simulink model "BatteryFastCharging"  (R2026a)
settings: Solver=ode23t  StopTime=p.Duration  MaxStep=1  RelTol=1e-5  AbsTol=1e-7
InitFcn:
  | addpath(fullfile(fileparts(get_param(bdroot,'FileName')),'matlab'));
model workspace (MAT data in the model file):
  logNames = {'time_s', 'current_charge_A', 'voltage_V', 'soc', 'core_K', 'surface_K', 'anode_potential_V', 'anode_surface_mol_m3', 'electrolyte_min_mol_m3', 'internal_soc', 'fault', 'sei_m', 'irreversible_plating_mol', 'reversible_plating_mol', 'complete', 'stop_after_settling', 'termination_reason', 'command_current_A', 'thermal_limit_A', 'anode_limit_A', 'electrolyte_limit_A', 'requested_current_A', 'binding_limiter', 'aging_enabled', 'characterization_replay'}
  p.Q_Ah = 5
  p.SOC0 = 0.2
  p.SOCtarget = 0.8
  p.T0 = 298.15
  p.Tamb = 298.15
  p.Vcontrol = 4.195
  p.Vmax = 4.2
  p.Tmax = 318.15
  p.Imax = 7.5
  p.AnodePotentialMin = 0.02
  p.ElectrolyteMin = 100
  p.Ts = 0.5
  p.Istages = [2.5 2.5 2.5 2.5]
  p.SOCswitch = [0.4 0.6 0.7]
  p.Duration = 12000
  p.Shells = 12
  p.LayersAnode = 12
  p.LayersSeparator = 12
  p.LayersCathode = 12
  p.UseExternalCurrent = 0
  p.InputCurrent = [0  0; 24000  0]
  p.EnableAging = 0
  p.InitialSEI = 5e-09
  p.CharacterizationReplay = 0
  p.StopOnTarget = 1
  p.ImaxDischarge = 7.5
  p.ActuatorTau = 2
  p.ThermalGain = 2
  p.ThermalSoftMargin = 1
  p.AnodeGain = 100
  p.AnodeFaultMin = -0.005
  p.ElectrolyteGain = 0.02
  p.ElectrolyteSoftMargin = 100
  p.VoltageFaultMargin = 0
  p.TemperatureFaultMargin = 0
  p.VoltageMin = 2
  p.SOCmin = 0
  p.DiagnosticVmax = 4.25
  p.DiagnosticVmin = 2
  p.DiagnosticTmax = 333.15
  p.DiagnosticCeMin = 1
  p.DiagnosticAnodeMin = -0.05
  p.ShutdownCurrentTolerance = 0.01
  p.ShutdownMinTime = 0.5
  p.ShutdownMaxTime = 20
  p.MaxStep = 1
  p.RelTol = 1e-05
  p.AbsTol = 1e-07
  p.RLsampleTime = 10
  p.ThicknessAnode = 8.52e-05
  p.ThicknessSeparator = 1.2e-05
  p.ThicknessCathode = 7.56e-05
  p.ElectrodePlateArea = 0.1027
  p.ParticleRadiusAnode = 5.86e-06
  p.ParticleRadiusCathode = 5.22e-06
  p.ActiveMaterialVolumeFractionAnode = 0.75
  p.ActiveMaterialVolumeFractionCathode = 0.665
  p.MaximumConcentrationAnode = 33133
  p.MaximumConcentrationCathode = 63104
  p.MinimumStoichiometryAnode = 0.0263457902706
  p.MaximumStoichiometryAnode = 0.910618046652
  p.MinimumStoichiometryCathode = 0.263845224591
  p.MaximumStoichiometryCathode = 0.85397467463
  p.ActiveMaterialDiffusionCoefficientAnode = 3.3e-14
  p.ActiveMaterialDiffusionCoefficientCathode = 4e-15
  p.ConductivityAnode = 215
  p.ConductivityCathode = 0.18
  p.CurrentCollectorResistance = 0
  p.ElectrolyteVolumeFractionAnode = 0.25
  p.ElectrolyteVolumeFractionSeparator = 0.47
  p.ElectrolyteVolumeFractionCathode = 0.335
  p.ElectrolyteConductivity = 0.9487
  p.ElectrolyteDiffusionCoefficient = 1.7694e-10
  p.BruggemanExponentAnode = 1.5
  p.BruggemanExponentSeparator = 1.5
  p.BruggemanExponentCathode = 1.5
  p.TransferenceNumber = 0.2594
  p.ChargeTransferRateAnode = 6.71604673749e-12
  p.ChargeTransferRateCathode = 3.54458022256e-11
  p.ArrheniusReferenceTemperature = 298.15
  p.ActiveMaterialDiffusionActivationEnergyAnode = 1e-06
  p.ActiveMaterialDiffusionActivationEnergyCathode = 1e-06
  p.ElectrolyteDiffusionActivationEnergy = 1e-06
  p.ElectrolyteConductivityActivationEnergy = 1e-06
  p.ConductivityActivationEnergyAnode = 1e-06
  p.ConductivityActivationEnergyCathode = 1e-06
  p.ChargeTransferActivationEnergyAnode = 35000
  p.ChargeTransferActivationEnergyCathode = 17800
  p.BatteryThermalMass = 42.7752981275
  p.Csurface = 8
  p.RcoreSurface = 1.5
  p.RsurfaceAmbient = 6
  p.Sto = [0.001 0.00266611018364 0.00433222036728 0.00599833055092 0.00766444073456 0.0093305509182 0.0109966611018 0.0126627712855 0.0143288814691 0.0159949916528 0.0176611018364 0.01932721202 ... (600 elements, 600x1)]
  p.Un = [2.30713653173 2.18632839865 2.07318676163 1.96722472974 1.86798629583 1.77504437364 1.68799895927 1.6064754091 1.53012282672 1.4586125519 1.39163674522 1.32890706202 ... (600 elements, 600x1)]
  p.Up = [4.67769531267 4.6763377305 4.67497967199 4.673621114 4.67226203229 4.67090240146 4.66954219491 4.66818138474 4.66681994175 4.66545783534 4.66409503344 4.66273150246 ... (600 elements, 600x1)]
  p.ProfileData = [0  2.5  2.5  2.5  2.5; 24000  2.5  2.5  2.5  2.5]
values from neighbouring files (symbols this model uses):
  p = project_parameters()    [additional_validation.m]    (also in aging_study.m = project_parameters();p.EnableAging=true; battery_diagnostics.m; build_report.m; evaluate_profile_selection.m)
libraries: fl_lib x6, nesl_utility x2, BatteryCurrentManagement x1, batt_lib x1
settings Model: Creator=venum  LastModifiedBy=venum

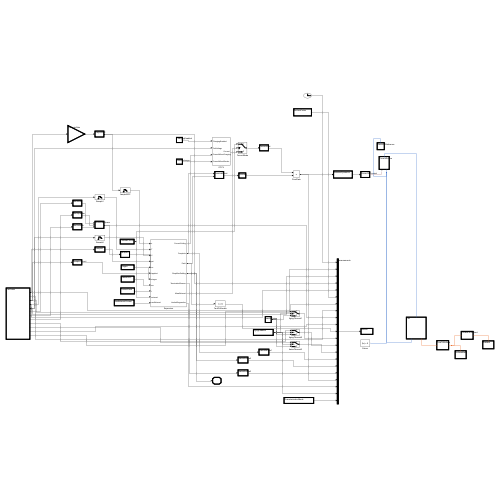
[thumbnail: Simulink's stored preview of the top-level diagram]
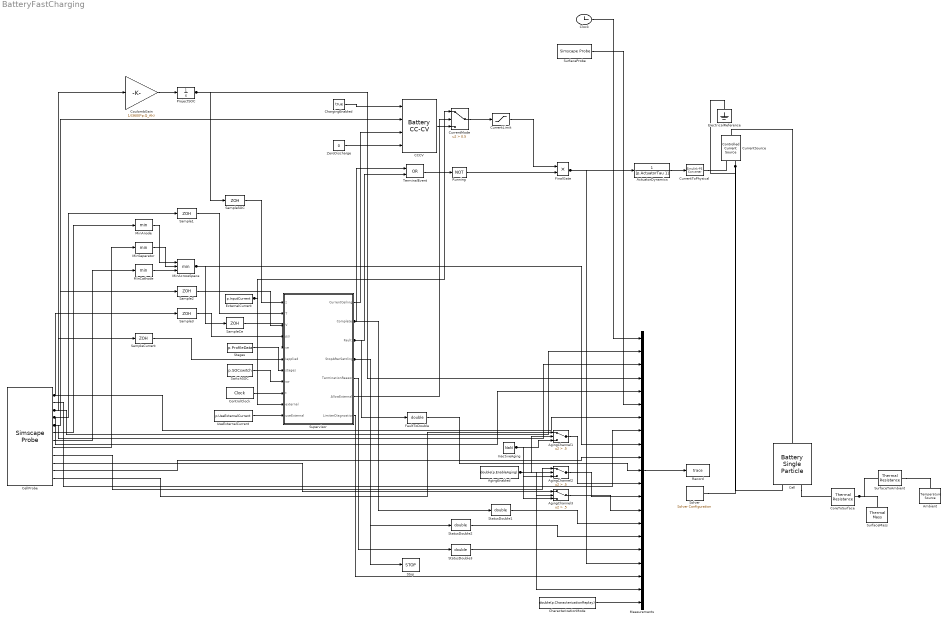
== system BatteryFastCharging ==
  ActuatorDynamics : TransferFcn  Numerator=1  Denominator=[p.ActuatorTau 1]
  AgingChannel1 : Switch  Criteria=u2 > Threshold  Threshold=.5  SaturateOnIntegerOverflow=off  InputSameDT=off
  AgingChannel2 : Switch  Criteria=u2 > Threshold  Threshold=.5  SaturateOnIntegerOverflow=off  InputSameDT=off
  AgingChannel3 : Switch  Criteria=u2 > Threshold  Threshold=.5  SaturateOnIntegerOverflow=off  InputSameDT=off
  AgingEnabled : Constant  Value=double(p.EnableAging)
  Ambient : fl_lib/Thermal/Thermal Sources/Temperature Source  temperature=p.Tamb K
  CCCV : BatteryCurrentManagement/Battery CC-CV  MinMaxFlag=off  MaxCellVoltage=p.Vcontrol  Kp=20  Ki=2  Kaw=1  Kt=1  Ts=p.Ts
  Cell : batt_lib/Cells/Electrochemical/Battery Single Particle  ExtrapolationMethod=simscape.enum.extrapolation.nearest  ThicknessAnode=p.ThicknessAnode m  ElectrolyteLayerCountAnode=p.LayersAnode  ThicknessSeparator=p.ThicknessSeparator m  ElectrolyteLayerCountSeparator=p.LayersSeparator  ThicknessCathode=p.ThicknessCathode m  ElectrolyteLayerCountCathode=p.LayersCathode  ElectrodePlateArea=p.ElectrodePlateArea m^2  ParticleRadiusAnode=p.ParticleRadiusAnode m  ShellCountAnode=p.Shells  ParticleRadiusCathode=p.ParticleRadiusCathode m  ShellCountCathode=p.Shells  ActiveMaterialVolumeFractionAnode=p.ActiveMaterialVolumeFractionAnode  ActiveMaterialVolumeFractionCathode=p.ActiveMaterialVolumeFractionCathode  StoichiometryBreakpointsSpecification=simscape.battery.enum.cells.electrochemical.StoichiometryBreakpointsSpecification.absolute  NormalizedStoichiometryBreakpoints=linspace(0.025, 0.975, 39)  OpenCircuitPotentialAnode=[.435; .325; .259; .221; .204; .194; .179; .166; .155; .145; .137; .131; .128; .127; .126; .125; .124; .123; .122; .121; .118; .117; .112; .109; .105; .1; .098; .095; .094; .093; .091; .09; .089; .088; .087; .086; .085; .084; .083] V  OpenCircuitPotentialCathode=[3.598; 3.53; 3.494; 3.474; 3.46; 3.455; 3.454; 3.453; 3.4528; 3.4526; 3.4524; 3.452; 3.4518; 3.4516; 3.4514; 3.4512; 3.451; 3.4508; 3.4506; 3.4503; 3.45; 3.4498; 3.4495; 3.4493; 3.449; 3.4488; 3.4486; 3.4484; 3.4482; 3.4479; 3.4477; 3.4475; 3.4473; 3.447; 3.4468; 3.4466; 3.4464; 3.4462; 3.4458] V  AbsoluteStoichiometryBreakpointsAnode=p.Sto  OpenCircuitPotentialAbsoluteAnode=p.Un V  AbsoluteStoichiometryBreakpointsCathode=p.Sto  OpenCircuitPotentialAbsoluteCathode=p.Up V  MaximumConcentrationAnode=p.MaximumConcentrationAnode mol/m^3  MaximumStoichiometryAnode=p.MaximumStoichiometryAnode  MinimumStoichiometryAnode=p.MinimumStoichiometryAnode  MaximumConcentrationCathode=p.MaximumConcentrationCathode mol/m^3  MaximumStoichiometryCathode=p.MaximumStoichiometryCathode  MinimumStoichiometryCathode=p.MinimumStoichiometryCathode  ActiveMaterialDiffusionCoefficientAnode=p.ActiveMaterialDiffusionCoefficientAnode m^2/s  ActiveMaterialDiffusionCoefficientCathode=p.ActiveMaterialDiffusionCoefficientCathode m^2/s  ConductivityAnode=p.ConductivityAnode S/m  ConductivityCathode=p.ConductivityCathode S/m  CurrentCollectorResistance=p.CurrentCollectorResistance Ohm  ElectrolyteVolumeFractionAnode=p.ElectrolyteVolumeFractionAnode  ElectrolyteVolumeFractionSeparator=p.ElectrolyteVolumeFractionSeparator  ElectrolyteVolumeFractionCathode=p.ElectrolyteVolumeFractionCathode  ElectrolyteConductivity=p.ElectrolyteConductivity S/m  BruggemanExponentAnode=p.BruggemanExponentAnode  BruggemanExponentSeparator=p.BruggemanExponentSeparator  BruggemanExponentCathode=p.BruggemanExponentCathode  TransferenceNumber=p.TransferenceNumber  ElectrolyteDiffusionCoefficient=p.ElectrolyteDiffusionCoefficient m^2/s  ChargeTransferRateAnode=p.ChargeTransferRateAnode m^(5/2)/(mol^(1/2)*s)  ChargeTransferRateCathode=p.ChargeTransferRateCathode m^(5/2)/(mol^(1/2)*s)  BatteryThermalMass=p.BatteryThermalMass J/K  ArrheniusReferenceTemperature=p.ArrheniusReferenceTemperature K  ActiveMaterialDiffusionActivationEnergyAnode=p.ActiveMaterialDiffusionActivationEnergyAnode J/mol  ActiveMaterialDiffusionActivationEnergyCathode=p.ActiveMaterialDiffusionActivationEnergyCathode J/mol  ElectrolyteDiffusionActivationEnergy=p.ElectrolyteDiffusionActivationEnergy J/mol  ConductivityActivationEnergyAnode=p.ConductivityActivationEnergyAnode J/mol  ConductivityActivationEnergyCathode=p.ConductivityActivationEnergyCathode J/mol  ElectrolyteConductivityActivationEnergy=p.ElectrolyteConductivityActivationEnergy J/mol  ChargeTransferActivationEnergyAnode=p.ChargeTransferActivationEnergyAnode J/mol  ChargeTransferActivationEnergyCathode=p.ChargeTransferActivationEnergyCathode J/mol  InnerSEIMethod=simscape.battery.enum.cells.electrochemical.InnerSEIMethod.none  MolarVolumeInnerSEI=9.585e-5 m^3/mol  DiffusionCoefficientInnerSEI=1e-20 m^2/s  StoichiometricCoefficientInnerSEI=2  DiffusionActivationEnergyInnerSEI=1e-6 J/mol  ConductivityInnerSEI=5e-6 S/m  ConductivityActivationEnergyInnerSEI=39000 J/mol  PlatingMethod=simscape.battery.enum.cells.electrochemical.PlatingMethod.none  ExchangeCurrentDensityPlating=3E-4 A/m^2  ActivationEnergyPlating=3000 J/mol  ReversibilityFactorPlating=0.5  batteryCurrent_specify=off  batteryCurrent_priority=None  batteryCurrent=0 A  batteryCurrent_nominal_specify=off  batteryCurrent_nominal_value=1  batteryCurrent_nominal_unit=A  batteryVoltage_specify=off  batteryVoltage_priority=None  batteryVoltage=0 V  batteryVoltage_nominal_specify=off  batteryVoltage_nominal_value=1  batteryVoltage_nominal_unit=V  averageElectrolyteConcentration_specify=on  averageElectrolyteConcentration_priority=High  averageElectrolyteConcentration=1000 mol/m^3  averageElectrolyteConcentration_nominal_specify=off  averageElectrolyteConcentration_nominal_value=1  averageElectrolyteConcentration_nominal_unit=mol/m^3  stateOfCharge_specify=on  stateOfCharge_priority=High  stateOfCharge=p.SOC0  stateOfCharge_nominal_specify=off  stateOfCharge_nominal_value=1  stateOfCharge_nominal_unit=1  batteryTemperature_specify=on  batteryTemperature_priority=High  batteryTemperature=p.T0 K  batteryTemperature_nominal_specify=off  batteryTemperature_nominal_value=1  batteryTemperature_nominal_unit=K  thicknessSEI_specify=on  thicknessSEI_priority=High  thicknessSEI=p.InitialSEI m  thicknessSEI_nominal_specify=off  thicknessSEI_nominal_value=1  thicknessSEI_nominal_unit=m  reversiblePlatedMaterial_specify=off  reversiblePlatedMaterial_priority=High  reversiblePlatedMaterial=0 mol  reversiblePlatedMaterial_nominal_specify=off  reversiblePlatedMaterial_nominal_value=1  reversiblePlatedMaterial_nominal_unit=mol  irreversiblePlatedMaterial_specify=off  irreversiblePlatedMaterial_priority=High  irreversiblePlatedMaterial=0 mol  irreversiblePlatedMaterial_nominal_specify=off  irreversiblePlatedMaterial_nominal_value=1  irreversiblePlatedMaterial_nominal_unit=mol  power_dissipated_specify=off  power_dissipated_priority=None  power_dissipated=0 W  power_dissipated_nominal_specify=off  power_dissipated_nominal_value=1  power_dissipated_nominal_unit=W  heatGenerationRate_specify=off  heatGenerationRate_priority=None  heatGenerationRate=0 W  heatGenerationRate_nominal_specify=off  heatGenerationRate_nominal_value=1  heatGenerationRate_nominal_unit=W
  CellProbe : SimscapeProbe  BoundBlock=1  Variables="{\"anodeElectrolyteOverpotential\":{\"Probing\":\"ON\"},\"anodeModel.surfaceConcentration\":{\"Probing\":\"ON\"},\"batteryCurrent\":{\"Probing\":\"ON\"},\"batteryTemperature\":{\"Probing\":\"ON\"},\"batteryVoltage\":{\"Probing\":\"ON\"},\"electrolyteModel.concentrationAnode\":{\"Probing\":\"ON\"},\"electrolyteModel.concentrationCathode\":{\"Probing\":\"ON\"},\"electrolyteModel.concentrationSeparator\":{\"Probing\":\"ON\"},\"irreversiblePlatedMaterial\":{\"Probing\":\"ON\"},\"reversiblePlatedMaterial\":{\"Probing\":\"ON\"},\"stateOfCharge\":{\"Probing\":\"ON\"},\"thicknessSEI\":{\"Probing\":\"ON\"}}"
  CharacterizationMode : Constant  Value=double(p.CharacterizationReplay)
  ChargingEnabled : Constant  Value=true  OutDataTypeStr=boolean
  Clock : Clock
  ControlClock : DigitalClock  SampleTime=p.Ts
  CoreToSurface : fl_lib/Thermal/Thermal Elements/Thermal Resistance  resistance=p.RcoreSurface K/W  T_specify=off  T_priority=None  T=0 K  T_nominal_specify=off  T_nominal_value=1  T_nominal_unit=K  Q_specify=off  Q_priority=None  Q=0 W  Q_nominal_specify=off  Q_nominal_value=1  Q_nominal_unit=W
  CoulombGain : Gain  Gain=1/(3600*p.Q_Ah)
  CurrentLimit : Saturate  UpperLimit=p.Imax  LowerLimit=-p.ImaxDischarge
  CurrentMode : Switch  Criteria=u2 > Threshold  Threshold=0.5  SaturateOnIntegerOverflow=off  InputSameDT=off
  CurrentSource : fl_lib/Electrical/Electrical Sources/Controlled Current Source
  CurrentToPhysical : nesl_utility/Simulink-PS Converter  PhysicalDomain=network_engine_domain  SubClassName=ps_input  LeftPortType=input  RightPortType=output  PseudoPeriodic=off  Frequencies=[]  NoiseDistribution=none  NoiseParameters=[]  Unit=A  AffineConversion=off  FilteringAndDerivatives=provide  SimscapeFilterOrder=1  InputFilterTimeConstant=0.001  UdotUserProvided=0
  ElectricalReference : fl_lib/Electrical/Electrical Elements/Electrical Reference
  ExternalCurrent : FromWorkspace  VariableName=p.InputCurrent  SampleTime=p.Ts
  FaultToDouble : DataTypeConversion  OutDataTypeStr=double  SaturateOnIntegerOverflow=off  RndMeth=Floor
  FinalGate : Product
  InactiveAging : Constant  Value=NaN
  Measurements : Mux  Inputs=21
  MinAcrossSpace : MinMax  Inputs=3
  MinAnode : MinMax
  MinCathode : MinMax
  MinSeparator : MinMax
  ProjectSOC : Integrator  InitialCondition=p.SOC0
  Record : ToWorkspace  VariableName=trace  SampleTime=-1
  Running : Logic  Operator=NOT  AllPortsSameDT=off  OutDataTypeStr=boolean
  Sample1 : ZeroOrderHold  SampleTime=p.Ts
  Sample2 : ZeroOrderHold  SampleTime=p.Ts
  Sample3 : ZeroOrderHold  SampleTime=p.Ts
  SampleCe : ZeroOrderHold  SampleTime=p.Ts
  SampleCurrent : ZeroOrderHold  SampleTime=p.Ts
  SampleSOC : ZeroOrderHold  SampleTime=p.Ts
  Solver : nesl_utility/Solver Configuration  PhysicalDomain=network_engine_domain  SubClassName=solver  LeftPortType=input  RightPortType=generic  Tones=[]  Harmonics=[]  SimulateNoise=off  Profile=off  UseLocalSampling=off  EnableSwitchedLinearOptims=on  FrequencyDomain=off  UseCCode=off  RelTol=0.001  AbsTol=0.001  MinStep=1e-09  ToWorkspace=off  RevertToSquareIcSolve=off  NumHomotopyIterations=100  PhasorMode=off  PhasorModeNumHarmonics=1  ConsistencySolver=NEWTON_XTOL_AFTER_FTOL  CanonicalOrdering=CANONICAL  OptimizeIntermediates=OPTIMIZED  IndexReductionMethod=DerivativeReplacement  DoDC=off  ResidualTolerance=1e-09  ConsistencyTolSource=GLOBAL  ConsistencyAbsTol=0.001  ConsistencyRelTol=0.001  ConsistencyTolFactor=0.001  UseLocalSolver=off  LocalSolverChoice=NE_BACKWARD_EULER_ADVANCER  ResolveIndetEquations=on  FunctionEvalNumThread=1  LocalSolverSampleTime=0.001  DoFixedCost=off  MaxNonlinIter=3  MaxModeIter=2  ComputeImpulses=off  ImpulseIterations=2  LinearAlgebra=auto  LinearAlgebraNumThread=0  EquationFormulation=NE_TIME_EF  DelaysMemoryBudget=1024  AutomaticFiltering=on  FilteringTimeConstant=0.001  PartitionStorageMethod=AS_NEEDED  PartitionMemoryBudget=1024  PartitionMethod=ROBUST  MultibodyUseLocalSolver=off  MultibodyLocalSolverChoice=ODE1  MultibodyLocalSolverSampleTime=0.001
  Stages : FromWorkspace  VariableName=p.ProfileData  SampleTime=p.Ts
  StatusDouble1 : DataTypeConversion  OutDataTypeStr=double  SaturateOnIntegerOverflow=off  RndMeth=Floor
  StatusDouble2 : DataTypeConversion  OutDataTypeStr=double  SaturateOnIntegerOverflow=off  RndMeth=Floor
  StatusDouble3 : DataTypeConversion  OutDataTypeStr=double  SaturateOnIntegerOverflow=off  RndMeth=Floor
  Stop : Stop
  Supervisor : Subsystem
  SurfaceMass : fl_lib/Thermal/Thermal Elements/Thermal Mass  mass_type=foundation.enum.constant_variable.constant  mass=1 kg  sp_heat=p.Csurface J/(K*kg)  mass_min=1e-6 kg  num_ports=foundation.enum.numPorts2.one  m_specify=off  m_priority=High  m=1 kg  m_nominal_specify=off  m_nominal_value=1  m_nominal_unit=kg  T_specify=on  T_priority=High  T=p.T0 K  T_nominal_specify=off  T_nominal_value=1  T_nominal_unit=K  Q_specify=off  Q_priority=None  Q=0 W  Q_nominal_specify=off  Q_nominal_value=1  Q_nominal_unit=W
  SurfaceProbe : SimscapeProbe  BoundBlock=8  Variables="{\"T\":{\"Probing\":\"ON\"}}"
  SurfaceToAmbient : fl_lib/Thermal/Thermal Elements/Thermal Resistance  resistance=p.RsurfaceAmbient K/W  T_specify=off  T_priority=None  T=0 K  T_nominal_specify=off  T_nominal_value=1  T_nominal_unit=K  Q_specify=off  Q_priority=None  Q=0 W  Q_nominal_specify=off  Q_nominal_value=1  Q_nominal_unit=W
  SwitchSOC : Constant  Value=p.SOCswitch
  TerminalEvent : Logic  Operator=OR  AllPortsSameDT=off  OutDataTypeStr=boolean
  UseExternalCurrent : Constant  Value=p.UseExternalCurrent
  ZeroDischarge : Constant  Value=0
  wires:
  CellProbe/8 -> MinSeparator/1
  CellProbe/1 -> Sample3/1, Measurements/7
  CellProbe/2 -> Measurements/8
  CellProbe/3 -> Measurements/2, CoulombGain/1, SampleCurrent/1
  CellProbe/4 -> Sample1/1, Measurements/5
  CellProbe/5 -> Sample2/1, CCCV/2, Measurements/3
  Supervisor/5(TerminationReason) -> StatusDouble3/1
  Sample2/1 -> Supervisor/3(V)
  CellProbe/6 -> MinAnode/1
  CellProbe/7 -> MinCathode/1
  AgingChannel1/1 -> Measurements/12
  CellProbe/9 -> AgingChannel2/1
  TerminalEvent/1 -> Running/1
  CellProbe/10 -> AgingChannel3/1
  Supervisor/2(Complete) -> StatusDouble1/1, TerminalEvent/1
  CellProbe/11 -> Measurements/10
  CellProbe/12 -> AgingChannel1/1
  CCCV/1 -> CurrentMode/3
  CoulombGain/1 -> ProjectSOC/1
  AgingChannel2/1 -> Measurements/13
  AgingEnabled/1 -> Measurements/20, AgingChannel1/2, AgingChannel2/2, AgingChannel3/2
  ExternalCurrent/1 -> CurrentMode/1, Supervisor/10(external)
  MinAnode/1 -> MinAcrossSpace/1
  MinSeparator/1 -> MinAcrossSpace/2
  MinCathode/1 -> MinAcrossSpace/3
  SampleCurrent/1 -> Supervisor/6(Iapplied)
  ProjectSOC/1 -> Measurements/4, SampleSOC/1
  Sample1/1 -> Supervisor/2(T)
  MinAcrossSpace/1 -> Measurements/9, SampleCe/1
  Supervisor/6(AllowExternal) -> CurrentMode/2
  Sample3/1 -> Supervisor/4(psi)
  ZeroDischarge/1 -> CCCV/4
  SampleSOC/1 -> Supervisor/1(z)
  SampleCe/1 -> Supervisor/5(ce)
  CurrentLimit/1 -> FinalGate/1
  Stages/1 -> Supervisor/7(stages)
  SwitchSOC/1 -> Supervisor/8(sw)
  ControlClock/1 -> Supervisor/9(t)
  UseExternalCurrent/1 -> Supervisor/11(useExternal)
  StatusDouble2/1 -> Measurements/16
  ChargingEnabled/1 -> CCCV/1
  Supervisor/1(CurrentCeiling) -> CCCV/3
  Clock/1 -> Measurements/1
  Supervisor/3(Fault) -> TerminalEvent/2, FaultToDouble/1
  Supervisor/4(StopAfterSettling) -> Stop/1, StatusDouble2/1
  Supervisor/7(LimiterDiagnostics) -> Measurements/19
  FaultToDouble/1 -> Measurements/11
  CurrentMode/1 -> CurrentLimit/1
  Running/1 -> FinalGate/2
  CharacterizationMode/1 -> Measurements/21
  StatusDouble3/1 -> Measurements/17
  InactiveAging/1 -> AgingChannel1/3, AgingChannel2/3, AgingChannel3/3
  StatusDouble1/1 -> Measurements/15
  SurfaceProbe/1 -> Measurements/6
  FinalGate/1 -> ActuatorDynamics/1, Measurements/18
  AgingChannel3/1 -> Measurements/14
  ActuatorDynamics/1 -> CurrentToPhysical/1
  Measurements/1 -> Record/1
  connections:
  CurrentToPhysical/RConn1 -- CurrentSource/RConn1
  CoreToSurface/RConn1 -- SurfaceMass/LConn1 -- SurfaceToAmbient/LConn1
  Cell/RConn2 -- CoreToSurface/LConn1
  CurrentSource/LConn1 -- Cell/LConn1
  Solver/RConn1 -- ElectricalReference/LConn1 -- Cell/RConn1 -- CurrentSource/RConn2
  SurfaceToAmbient/RConn1 -- Ambient/LConn1

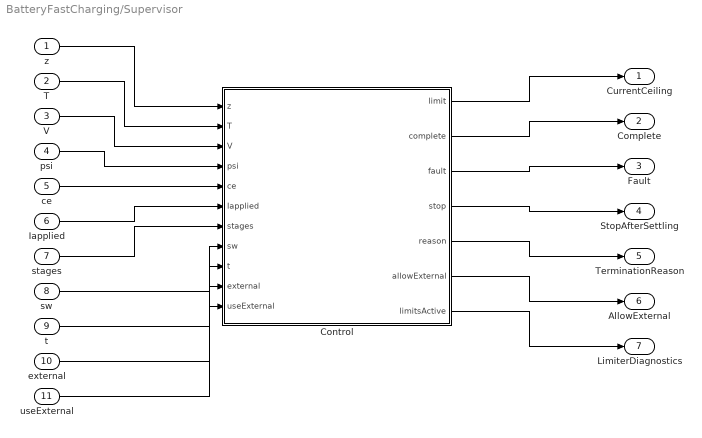
== system BatteryFastCharging/Supervisor ==
  z : Inport
  T : Inport  Port=2
  V : Inport  Port=3
  psi : Inport  Port=4
  ce : Inport  Port=5
  Iapplied : Inport  Port=6
  stages : Inport  Port=7
  sw : Inport  Port=8
  t : Inport  Port=9
  external : Inport  Port=10
  useExternal : Inport  Port=11
  Control : MATLAB Function  TreatAsAtomicUnit=on
  CurrentCeiling : Outport
  Complete : Outport  Port=2
  Fault : Outport  Port=3
  StopAfterSettling : Outport  Port=4
  TerminationReason : Outport  Port=5
  AllowExternal : Outport  Port=6
  LimiterDiagnostics : Outport  Port=7
  wires:
  z/1 -> Control/1(z)
  T/1 -> Control/2(T)
  V/1 -> Control/3(V)
  psi/1 -> Control/4(psi)
  ce/1 -> Control/5(ce)
  Iapplied/1 -> Control/6(Iapplied)
  stages/1 -> Control/7(stages)
  sw/1 -> Control/8(sw)
  t/1 -> Control/9(t)
  external/1 -> Control/10(external)
  useExternal/1 -> Control/11(useExternal)
  Control/1(limit) -> CurrentCeiling/1
  Control/2(complete) -> Complete/1
  Control/3(fault) -> Fault/1
  Control/4(stop) -> StopAfterSettling/1
  Control/5(reason) -> TerminationReason/1
  Control/6(allowExternal) -> AllowExternal/1
  Control/7(limitsActive) -> LimiterDiagnostics/1

== matlab function BatteryFastCharging/Supervisor/Control ==
  data: z input; limit output; T input; V input; psi input; ce input; Iapplied input; stages input; sw input; t input; external input; useExternal input; complete output; fault output; stop output; reason output; allowExternal output; limitsActive output; p parameter
function [limit,complete,fault,stop,reason,allowExternal,limitsActive]=supervisor_step(z,T,V,psi,ce,Iapplied,stages,sw,t,external,useExternal,p)
%#codegen
% Named states and parameters; reasons are latched through shutdown settling.
% 0 running; 1 completed; 2 V high; 3 T high; 4 anode; 5 electrolyte;
% 6 V low/SOC low; 7 nonfinite measurement. Postprocessor adds 8 timeout.
persistent eventCode eventTime
if isempty(eventCode),eventCode=0;eventTime=0;end
if z<sw(1),requested=stages(1);
elseif z<sw(2),requested=stages(2);
elseif z<sw(3),requested=stages(3);
else,requested=stages(4);end
if useExternal>0.5,requested=external;end
thermal=p.ThermalGain*max(0,p.Tmax-p.ThermalSoftMargin-T);
anode=p.AnodeGain*max(0,psi-p.AnodePotentialMin);
electrolyte=p.ElectrolyteGain*max(0,ce-p.ElectrolyteMin-p.ElectrolyteSoftMargin);
limit=max(0,min([requested,p.Imax,thermal,anode,electrolyte]));
binding=0;
if requested>0,[~,binding]=min([requested,p.Imax,thermal,anode,electrolyte]);end
diagnostic=p.CharacterizationReplay && useExternal>0.5;
allowExternal=useExternal>0.5 && (diagnostic || requested<0);
vmax=p.Vmax+p.VoltageFaultMargin;tmax=p.Tmax+p.TemperatureFaultMargin;
vmin=p.VoltageMin;cefloor=p.ElectrolyteMin;psifloor=p.AnodeFaultMin;
if diagnostic
 vmax=p.DiagnosticVmax;vmin=p.DiagnosticVmin;tmax=p.DiagnosticTmax;
 cefloor=p.DiagnosticCeMin;psifloor=p.DiagnosticAnodeMin;
 limit=max(0,min(requested,p.Imax));binding=0;
end
newCode=0;
if ~all(isfinite([z,T,V,psi,ce,Iapplied])),newCode=7;
elseif V>vmax,newCode=2;
elseif T>tmax,newCode=3;
elseif psi<psifloor,newCode=4;
elseif ce<cefloor,newCode=5;
elseif V<vmin || z<p.SOCmin-1e-3,newCode=6;
elseif p.StopOnTarget && z>=p.SOCtarget,newCode=1;
end
if eventCode==0 && newCode>0,eventCode=newCode;eventTime=t;
elseif eventCode==1 && newCode>1,eventCode=newCode;end
reason=eventCode;complete=eventCode==1;fault=eventCode>1;
if eventCode>0,limit=0;end
settled=abs(Iapplied)<=p.ShutdownCurrentTolerance && t-eventTime>=p.ShutdownMinTime;
stop=eventCode>0 && (settled || t-eventTime>=p.ShutdownMaxTime);
limitsActive=[thermal;anode;electrolyte;requested;binding];
end
